simulink model "NUgus_contact"  (R2018a)
settings: Solver=VariableStepAuto  StartTime=0.0  StopTime=inf  RelTol=1e-3
values from neighbouring files (symbols this model uses):
  h_pitch = 0    [init.m]    (also in zombie.m)
  h_yaw = 0    [init.m]    (also in zombie.m)
  head = [-0.05482228998067195, -0.00010888238321339966, 0.0011712900228573724, 0.41900000000000004]    [comtest.m]
  l_ankle_pitch = 0    [init.m]    (also in zombie.m)
  l_ankle_roll = 0    [init.m]    (also in zombie.m)
  l_elbow_pitch = 0    [init.m]    (also in zombie.m)
  l_hip_pitch = 0    [init.m]    (also in zombie.m)
  l_hip_roll = 0    [init.m]    (also in zombie.m)
  l_hip_yaw = 0    [init.m]    (also in zombie.m)
  l_knee_pitch = 0    [init.m]    (also in zombie.m)
  l_shoulder_pitch = 0    [init.m]    (also in zombie.m)
  l_shoulder_roll = 0    [init.m]    (also in zombie.m)
  r_ankle_pitch = 0    [init.m]    (also in zombie.m)
  r_ankle_roll = 0    [init.m]    (also in zombie.m)
  r_elbow_pitch = 0    [init.m]    (also in zombie.m)
  r_hip_pitch = 0    [init.m]    (also in zombie.m)
  r_hip_roll = 0    [init.m]    (also in zombie.m)
  r_hip_yaw = 0    [init.m]    (also in zombie.m)
  r_knee_pitch = 0    [init.m]    (also in zombie.m)
  r_shoulder_pitch = 0    [init.m]    (also in zombie.m)
  r_shoulder_roll = 0    [init.m]    (also in zombie.m)
  s = mean(abs(present_speed.data))    [RunServoTest.m]
  torso = [0.0050079703254699804, 0.008880921777563762, 0.1021503146237477, 2.5390000000000006]    [comtest.m]
undefined symbols (not defined in the file or in its folder): floor, X, Y, Z
libraries: sm_lib x206, fl_lib x128, nesl_utility x21
(part 6 of 6)

== system NUgus_contact/right_foot/foot_fr_contact ==
  6-DOF Joint : sm_lib/Joints/6-DOF Joint  SenseConstraintForce=off  SenseConstraintForceX=off  SenseConstraintForceY=off  SenseConstraintForceZ=off  SenseConstraintTorque=off  SenseConstraintTorqueX=off  SenseConstraintTorqueY=off  SenseConstraintTorqueZ=off  SenseTotalForce=off  SenseTotalForceX=off  SenseTotalForceY=off  SenseTotalForceZ=off  SenseTotalTorque=off  SenseTotalTorqueX=off  SenseTotalTorqueY=off  SenseTotalTorqueZ=off  CompositeWrenchDir=FollowerOnBase  CompositeWrenchFrame=BaseFrame  PxEquilibriumPosition=0  PxEquilibriumPositionUnits=m  PxSpringStiffness=0  PxSpringStiffnessUnits=N/m  PxDampingCoefficient=0  PxDampingCoefficientUnits=N/(m/s)  PxTorqueActuationMode=InputTorque  PxMotionActuationMode=ComputedMotion  PxSensePosition=off  PxSenseVelocity=on  PxSenseAcceleration=off  PxSenseTorqueForce=off  PxPositionTargetSpecify=off  PxPositionTargetPriority=High  PxPositionTargetValue=0  PxPositionTargetValueUnits=m  PxVelocityTargetSpecify=off  PxVelocityTargetPriority=High  PxVelocityTargetValue=0  PxVelocityTargetValueUnits=m/s  PyEquilibriumPosition=0  PyEquilibriumPositionUnits=m  PySpringStiffness=0  PySpringStiffnessUnits=N/m  PyDampingCoefficient=0  PyDampingCoefficientUnits=N/(m/s)  PyTorqueActuationMode=InputTorque  PyMotionActuationMode=ComputedMotion  PySensePosition=off  PySenseVelocity=on  PySenseAcceleration=off  PySenseTorqueForce=off  PyPositionTargetSpecify=off  PyPositionTargetPriority=High  PyPositionTargetValue=0  PyPositionTargetValueUnits=m  PyVelocityTargetSpecify=off  PyVelocityTargetPriority=High  PyVelocityTargetValue=0  PyVelocityTargetValueUnits=m/s  PzEquilibriumPosition=0  PzEquilibriumPositionUnits=m  PzSpringStiffness=0  PzSpringStiffnessUnits=N/m  PzDampingCoefficient=0  PzDampingCoefficientUnits=N/(m/s)  PzTorqueActuationMode=InputTorque  PzMotionActuationMode=ComputedMotion  PzSensePosition=on  PzSenseVelocity=on  PzSenseAcceleration=off  PzSenseTorqueForce=off  PzPositionTargetSpecify=off  PzPositionTargetPriority=High  PzPositionTargetValue=0  PzPositionTargetValueUnits=m  PzVelocityTargetSpecify=off  PzVelocityTargetPriority=High  PzVelocityTargetValue=0  PzVelocityTargetValueUnits=m/s  SphDefPosRotationMethod=None  SphDefPosRotationAngleUnits=deg  SphDefPosRotationStandardAxis=+Z  SphDefPosRotationAngle=0.0  SphDefPosRotationArbitraryAxis=[0 0 1]  SphDefPosFollAlignAxisA=+X  SphDefPosBaseAlignAxisA=+Y  SphDefPosFollAlignAxisB=+Y  SphDefPosBaseAlignAxisB=+Z  SphDefPosRotationSequenceAxes=FollowerAxes  SphDefPosRotationSequence=XYX  SphDefPosRotationSequenceAngles=[0 0 0]  SphDefPosRotationSequenceAnglesUnits=deg  SphDefPosRotationMatrix=[1 0 0; 0 1 0; 0 0 1]  SphEqPosRotationMethod=None  SphEqPosRotationAngleUnits=deg  SphEqPosRotationStandardAxis=+Z  SphEqPosRotationAngle=0.0  SphEqPosRotationArbitraryAxis=[0 0 1]  SphEqPosFollAlignAxisA=+X  SphEqPosBaseAlignAxisA=+Y  SphEqPosFollAlignAxisB=+Y  SphEqPosBaseAlignAxisB=+Z  SphEqPosRotationSequenceAxes=FollowerAxes  SphEqPosRotationSequence=XYX  SphEqPosRotationSequenceAngles=[0 0 0]  SphEqPosRotationSequenceAnglesUnits=deg  SphEqPosRotationMatrix=[1 0 0; 0 1 0; 0 0 1]  SphSpringStiffness=0  SphSpringStiffnessUnits=N*m/deg  SphDampingCoefficient=0  SphDampingCoefficientUnits=N*m/(deg/s)  SphActuateTorqueX=off  SphActuateTorqueY=off  SphActuateTorqueZ=off  SphActuateTorque=off  SphTorqueActuationMode=NoTorque  SphMotionActuationMode=ComputedMotion  SphActuationFrame=BaseFrame  SphSensePosition=off  SphSenseVelocityX=off  SphSenseVelocityY=off  SphSenseVelocityZ=off  SphSenseVelocity=off  SphSenseAccelerationX=off  SphSenseAccelerationY=off  SphSenseAccelerationZ=off  SphSenseAcceleration=off  SphSenseTorqueX=off  SphSenseTorqueY=off  SphSenseTorqueZ=off  SphSenseTorqueForce=off  SphSensingFrame=BaseFrame  SphPositionTargetRotationMethod=None  SphPositionTargetRotationAngleUnits=deg  SphPositionTargetRotationStandardAxis=+Z  SphPositionTargetRotationAngle=0.0  SphPositionTargetRotationArbitraryAxis=[0 0 1]  SphPositionTargetFollAlignAxisA=+X  SphPositionTargetBaseAlignAxisA=+Y  SphPositionTargetFollAlignAxisB=+Y  SphPositionTargetBaseAlignAxisB=+Z  SphPositionTargetRotationSequenceAxes=FollowerAxes  SphPositionTargetRotationSequence=XYX  SphPositionTargetRotationSequenceAngles=[0 0 0]  SphPositionTargetRotationSequenceAnglesUnits=deg  SphPositionTargetRotationMatrix=[1 0 0; 0 1 0; 0 0 1]  SphPositionTargetSpecify=off  SphPositionTargetPriority=High  SphVelocityTargetValue=[0 0 0]  SphVelocityTargetValueUnits=deg/s  SphVelocityTargetSpecify=off  SphVelocityTargetPriority=High  SphVelocityTargetInFollowerFrame=on
  PS Abs : fl_lib/Physical Signals/Nonlinear Operators/PS Abs
      settings: SourceProductName=Simscape  SourceProductBaseCode=SS
  calculate forces : Subsystem
  friction gain : fl_lib/Physical Signals/Functions/PS Gain  gain=floor.friction
  x Velocity Gain : fl_lib/Physical Signals/Functions/PS Gain  gain=floor.vel_gain
  y Velocity Gain : fl_lib/Physical Signals/Functions/PS Gain  gain=floor.vel_gain
  z Position gain : fl_lib/Physical Signals/Functions/PS Gain  gain=floor.pos_gain
  z Velocity Gain : fl_lib/Physical Signals/Functions/PS Gain  gain=floor.vel_gain
  z add : fl_lib/Physical Signals/Functions/PS Add
  Contact : PMIOPort  Side=Right
  Floor : PMIOPort  Port=2  Side=Left
  connections:
  6-DOF Joint/RConn1 -- Contact/RConn1
  Floor/RConn1 -- 6-DOF Joint/LConn1
  6-DOF Joint/RConn4 -- calculate forces/LConn3 -- z Position gain/LConn1
  z Velocity Gain/LConn1 -- 6-DOF Joint/RConn5
  y Velocity Gain/LConn1 -- 6-DOF Joint/RConn3
  x Velocity Gain/LConn1 -- 6-DOF Joint/RConn2
  z Position gain/RConn1 -- z add/LConn1
  z Velocity Gain/RConn1 -- z add/LConn2
  PS Abs/LConn1 -- friction gain/RConn1
  z add/RConn1 -- friction gain/LConn1 -- calculate forces/LConn4
  calculate forces/LConn1 -- x Velocity Gain/RConn1
  calculate forces/LConn2 -- y Velocity Gain/RConn1
  calculate forces/LConn5 -- PS Abs/RConn1
  calculate forces/RConn1 -- 6-DOF Joint/LConn2
  calculate forces/RConn2 -- 6-DOF Joint/LConn3
  calculate forces/RConn3 -- 6-DOF Joint/LConn4

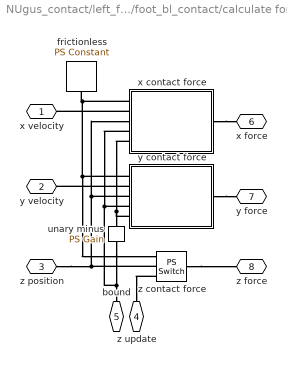
== system NUgus_contact/left_foot/foot_bl_contact/calculate forces ==
  frictionless : fl_lib/Physical Signals/Sources/PS Constant  constant=0
  unary minus : fl_lib/Physical Signals/Functions/PS Gain  gain=-1
  x contact force : Subsystem
  y contact force : Subsystem
  z contact force : fl_lib/Physical Signals/Nonlinear Operators/PS Switch  Threshold=0
      settings: SourceProductName=Simscape  SourceProductBaseCode=SS
  x velocity : PMIOPort  Side=Left
  y velocity : PMIOPort  Port=2  Side=Left
  z position : PMIOPort  Port=3  Side=Left
  z update : PMIOPort  Port=4  Side=Left
  bound : PMIOPort  Port=5  Side=Left
  x force : PMIOPort  Port=6  Side=Right
  y force : PMIOPort  Port=7  Side=Right
  z force : PMIOPort  Port=8  Side=Right
  connections:
  x contact force/LConn2 -- x velocity/RConn1
  y contact force/LConn2 -- y velocity/RConn1
  y contact force/RConn1 -- y force/RConn1
  x contact force/RConn1 -- x force/RConn1
  z contact force/RConn1 -- z force/RConn1
  y contact force/LConn3 -- x contact force/LConn3 -- z position/RConn1 -- z contact force/LConn2
  y contact force/LConn4 -- x contact force/LConn4 -- unary minus/LConn1 -- bound/RConn1
  y contact force/LConn5 -- x contact force/LConn5 -- unary minus/RConn1
  x contact force/LConn1 -- frictionless/RConn1 -- y contact force/LConn1 -- z contact force/LConn1
  z contact force/LConn3 -- z update/RConn1

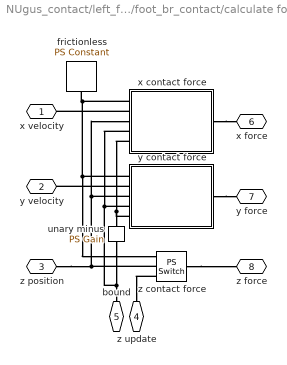
== system NUgus_contact/left_foot/foot_br_contact/calculate forces ==
  frictionless : fl_lib/Physical Signals/Sources/PS Constant  constant=0
  unary minus : fl_lib/Physical Signals/Functions/PS Gain  gain=-1
  x contact force : Subsystem
  y contact force : Subsystem
  z contact force : fl_lib/Physical Signals/Nonlinear Operators/PS Switch  Threshold=0
      settings: SourceProductName=Simscape  SourceProductBaseCode=SS
  x velocity : PMIOPort  Side=Left
  y velocity : PMIOPort  Port=2  Side=Left
  z position : PMIOPort  Port=3  Side=Left
  z update : PMIOPort  Port=4  Side=Left
  bound : PMIOPort  Port=5  Side=Left
  x force : PMIOPort  Port=6  Side=Right
  y force : PMIOPort  Port=7  Side=Right
  z force : PMIOPort  Port=8  Side=Right
  connections:
  x contact force/LConn2 -- x velocity/RConn1
  y contact force/LConn2 -- y velocity/RConn1
  y contact force/RConn1 -- y force/RConn1
  x contact force/RConn1 -- x force/RConn1
  z contact force/RConn1 -- z force/RConn1
  y contact force/LConn3 -- x contact force/LConn3 -- z position/RConn1 -- z contact force/LConn2
  y contact force/LConn4 -- x contact force/LConn4 -- unary minus/LConn1 -- bound/RConn1
  y contact force/LConn5 -- x contact force/LConn5 -- unary minus/RConn1
  x contact force/LConn1 -- frictionless/RConn1 -- y contact force/LConn1 -- z contact force/LConn1
  z contact force/LConn3 -- z update/RConn1

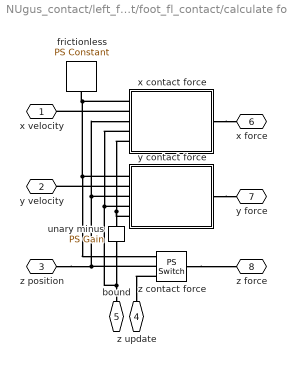
== system NUgus_contact/left_foot/foot_fl_contact/calculate forces ==
  frictionless : fl_lib/Physical Signals/Sources/PS Constant  constant=0
  unary minus : fl_lib/Physical Signals/Functions/PS Gain  gain=-1
  x contact force : Subsystem
  y contact force : Subsystem
  z contact force : fl_lib/Physical Signals/Nonlinear Operators/PS Switch  Threshold=0
      settings: SourceProductName=Simscape  SourceProductBaseCode=SS
  x velocity : PMIOPort  Side=Left
  y velocity : PMIOPort  Port=2  Side=Left
  z position : PMIOPort  Port=3  Side=Left
  z update : PMIOPort  Port=4  Side=Left
  bound : PMIOPort  Port=5  Side=Left
  x force : PMIOPort  Port=6  Side=Right
  y force : PMIOPort  Port=7  Side=Right
  z force : PMIOPort  Port=8  Side=Right
  connections:
  x contact force/LConn2 -- x velocity/RConn1
  y contact force/LConn2 -- y velocity/RConn1
  y contact force/RConn1 -- y force/RConn1
  x contact force/RConn1 -- x force/RConn1
  z contact force/RConn1 -- z force/RConn1
  y contact force/LConn3 -- x contact force/LConn3 -- z position/RConn1 -- z contact force/LConn2
  y contact force/LConn4 -- x contact force/LConn4 -- unary minus/LConn1 -- bound/RConn1
  y contact force/LConn5 -- x contact force/LConn5 -- unary minus/RConn1
  x contact force/LConn1 -- frictionless/RConn1 -- y contact force/LConn1 -- z contact force/LConn1
  z contact force/LConn3 -- z update/RConn1

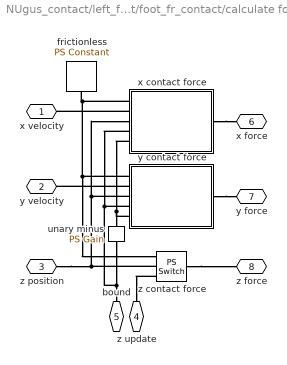
== system NUgus_contact/left_foot/foot_fr_contact/calculate forces ==
  frictionless : fl_lib/Physical Signals/Sources/PS Constant  constant=0
  unary minus : fl_lib/Physical Signals/Functions/PS Gain  gain=-1
  x contact force : Subsystem
  y contact force : Subsystem
  z contact force : fl_lib/Physical Signals/Nonlinear Operators/PS Switch  Threshold=0
      settings: SourceProductName=Simscape  SourceProductBaseCode=SS
  x velocity : PMIOPort  Side=Left
  y velocity : PMIOPort  Port=2  Side=Left
  z position : PMIOPort  Port=3  Side=Left
  z update : PMIOPort  Port=4  Side=Left
  bound : PMIOPort  Port=5  Side=Left
  x force : PMIOPort  Port=6  Side=Right
  y force : PMIOPort  Port=7  Side=Right
  z force : PMIOPort  Port=8  Side=Right
  connections:
  x contact force/LConn2 -- x velocity/RConn1
  y contact force/LConn2 -- y velocity/RConn1
  y contact force/RConn1 -- y force/RConn1
  x contact force/RConn1 -- x force/RConn1
  z contact force/RConn1 -- z force/RConn1
  y contact force/LConn3 -- x contact force/LConn3 -- z position/RConn1 -- z contact force/LConn2
  y contact force/LConn4 -- x contact force/LConn4 -- unary minus/LConn1 -- bound/RConn1
  y contact force/LConn5 -- x contact force/LConn5 -- unary minus/RConn1
  x contact force/LConn1 -- frictionless/RConn1 -- y contact force/LConn1 -- z contact force/LConn1
  z contact force/LConn3 -- z update/RConn1

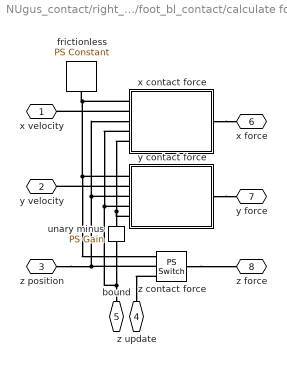
== system NUgus_contact/right_foot/foot_bl_contact/calculate forces ==
  frictionless : fl_lib/Physical Signals/Sources/PS Constant  constant=0
  unary minus : fl_lib/Physical Signals/Functions/PS Gain  gain=-1
  x contact force : Subsystem
  y contact force : Subsystem
  z contact force : fl_lib/Physical Signals/Nonlinear Operators/PS Switch  Threshold=0
      settings: SourceProductName=Simscape  SourceProductBaseCode=SS
  x velocity : PMIOPort  Side=Left
  y velocity : PMIOPort  Port=2  Side=Left
  z position : PMIOPort  Port=3  Side=Left
  z update : PMIOPort  Port=4  Side=Left
  bound : PMIOPort  Port=5  Side=Left
  x force : PMIOPort  Port=6  Side=Right
  y force : PMIOPort  Port=7  Side=Right
  z force : PMIOPort  Port=8  Side=Right
  connections:
  x contact force/LConn2 -- x velocity/RConn1
  y contact force/LConn2 -- y velocity/RConn1
  y contact force/RConn1 -- y force/RConn1
  x contact force/RConn1 -- x force/RConn1
  z contact force/RConn1 -- z force/RConn1
  y contact force/LConn3 -- x contact force/LConn3 -- z position/RConn1 -- z contact force/LConn2
  y contact force/LConn4 -- x contact force/LConn4 -- unary minus/LConn1 -- bound/RConn1
  y contact force/LConn5 -- x contact force/LConn5 -- unary minus/RConn1
  x contact force/LConn1 -- frictionless/RConn1 -- y contact force/LConn1 -- z contact force/LConn1
  z contact force/LConn3 -- z update/RConn1

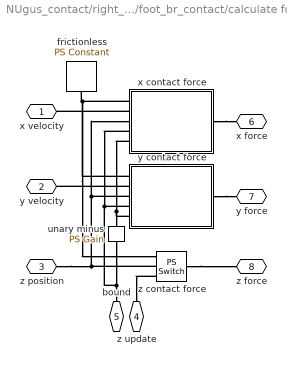
== system NUgus_contact/right_foot/foot_br_contact/calculate forces ==
  frictionless : fl_lib/Physical Signals/Sources/PS Constant  constant=0
  unary minus : fl_lib/Physical Signals/Functions/PS Gain  gain=-1
  x contact force : Subsystem
  y contact force : Subsystem
  z contact force : fl_lib/Physical Signals/Nonlinear Operators/PS Switch  Threshold=0
      settings: SourceProductName=Simscape  SourceProductBaseCode=SS
  x velocity : PMIOPort  Side=Left
  y velocity : PMIOPort  Port=2  Side=Left
  z position : PMIOPort  Port=3  Side=Left
  z update : PMIOPort  Port=4  Side=Left
  bound : PMIOPort  Port=5  Side=Left
  x force : PMIOPort  Port=6  Side=Right
  y force : PMIOPort  Port=7  Side=Right
  z force : PMIOPort  Port=8  Side=Right
  connections:
  x contact force/LConn2 -- x velocity/RConn1
  y contact force/LConn2 -- y velocity/RConn1
  y contact force/RConn1 -- y force/RConn1
  x contact force/RConn1 -- x force/RConn1
  z contact force/RConn1 -- z force/RConn1
  z contact force/LConn2 -- z position/RConn1 -- y contact force/LConn3 -- x contact force/LConn3
  unary minus/LConn1 -- y contact force/LConn4 -- x contact force/LConn4 -- bound/RConn1
  x contact force/LConn5 -- y contact force/LConn5 -- unary minus/RConn1
  x contact force/LConn1 -- y contact force/LConn1 -- z contact force/LConn1 -- frictionless/RConn1
  z contact force/LConn3 -- z update/RConn1

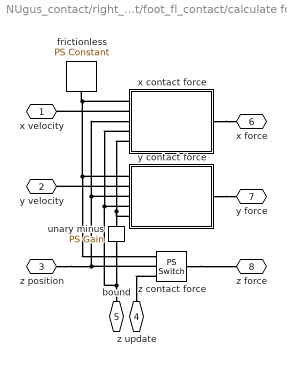
== system NUgus_contact/right_foot/foot_fl_contact/calculate forces ==
  frictionless : fl_lib/Physical Signals/Sources/PS Constant  constant=0
  unary minus : fl_lib/Physical Signals/Functions/PS Gain  gain=-1
  x contact force : Subsystem
  y contact force : Subsystem
  z contact force : fl_lib/Physical Signals/Nonlinear Operators/PS Switch  Threshold=0
      settings: SourceProductName=Simscape  SourceProductBaseCode=SS
  x velocity : PMIOPort  Side=Left
  y velocity : PMIOPort  Port=2  Side=Left
  z position : PMIOPort  Port=3  Side=Left
  z update : PMIOPort  Port=4  Side=Left
  bound : PMIOPort  Port=5  Side=Left
  x force : PMIOPort  Port=6  Side=Right
  y force : PMIOPort  Port=7  Side=Right
  z force : PMIOPort  Port=8  Side=Right
  connections:
  x contact force/LConn2 -- x velocity/RConn1
  y contact force/LConn2 -- y velocity/RConn1
  y contact force/RConn1 -- y force/RConn1
  x contact force/RConn1 -- x force/RConn1
  z contact force/RConn1 -- z force/RConn1
  y contact force/LConn3 -- x contact force/LConn3 -- z position/RConn1 -- z contact force/LConn2
  y contact force/LConn4 -- x contact force/LConn4 -- unary minus/LConn1 -- bound/RConn1
  y contact force/LConn5 -- x contact force/LConn5 -- unary minus/RConn1
  x contact force/LConn1 -- frictionless/RConn1 -- y contact force/LConn1 -- z contact force/LConn1
  z contact force/LConn3 -- z update/RConn1

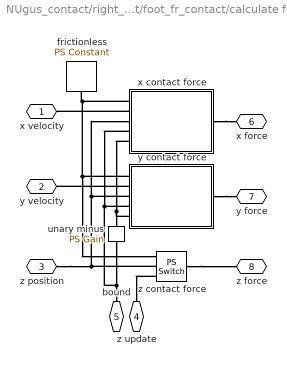
== system NUgus_contact/right_foot/foot_fr_contact/calculate forces ==
  frictionless : fl_lib/Physical Signals/Sources/PS Constant  constant=0
  unary minus : fl_lib/Physical Signals/Functions/PS Gain  gain=-1
  x contact force : Subsystem
  y contact force : Subsystem
  z contact force : fl_lib/Physical Signals/Nonlinear Operators/PS Switch  Threshold=0
      settings: SourceProductName=Simscape  SourceProductBaseCode=SS
  x velocity : PMIOPort  Side=Left
  y velocity : PMIOPort  Port=2  Side=Left
  z position : PMIOPort  Port=3  Side=Left
  z update : PMIOPort  Port=4  Side=Left
  bound : PMIOPort  Port=5  Side=Left
  x force : PMIOPort  Port=6  Side=Right
  y force : PMIOPort  Port=7  Side=Right
  z force : PMIOPort  Port=8  Side=Right
  connections:
  x contact force/LConn2 -- x velocity/RConn1
  y contact force/LConn2 -- y velocity/RConn1
  y contact force/RConn1 -- y force/RConn1
  x contact force/RConn1 -- x force/RConn1
  z contact force/RConn1 -- z force/RConn1
  y contact force/LConn3 -- x contact force/LConn3 -- z position/RConn1 -- z contact force/LConn2
  y contact force/LConn4 -- x contact force/LConn4 -- unary minus/LConn1 -- bound/RConn1
  y contact force/LConn5 -- x contact force/LConn5 -- unary minus/RConn1
  x contact force/LConn1 -- frictionless/RConn1 -- y contact force/LConn1 -- z contact force/LConn1
  z contact force/LConn3 -- z update/RConn1

== system NUgus_contact/left_foot/foot_bl_contact/calculate forces/x contact force ==
  PS Max : fl_lib/Physical Signals/Nonlinear Operators/PS Max
      settings: SourceProductName=Simscape  SourceProductBaseCode=SS
  PS Min : fl_lib/Physical Signals/Nonlinear Operators/PS Min
      settings: SourceProductName=Simscape  SourceProductBaseCode=SS
  PS Switch1 : fl_lib/Physical Signals/Nonlinear Operators/PS Switch  Threshold=0
      settings: SourceProductName=Simscape  SourceProductBaseCode=SS
  frictionless : PMIOPort  Side=Left
  force : PMIOPort  Port=2  Side=Right
  velocity : PMIOPort  Port=3  Side=Left
  z position : PMIOPort  Port=4  Side=Left
  upper_bound : PMIOPort  Port=5  Side=Left
  lower_bound : PMIOPort  Port=6  Side=Left
  connections:
  PS Max/LConn2 -- lower_bound/RConn1
  PS Max/LConn1 -- PS Min/RConn1
  PS Switch1/LConn3 -- PS Max/RConn1
  PS Min/LConn1 -- velocity/RConn1
  z position/RConn1 -- PS Switch1/LConn2
  PS Switch1/LConn1 -- frictionless/RConn1
  PS Switch1/RConn1 -- force/RConn1
  PS Min/LConn2 -- upper_bound/RConn1

== system NUgus_contact/left_foot/foot_bl_contact/calculate forces/y contact force ==
  PS Max : fl_lib/Physical Signals/Nonlinear Operators/PS Max
      settings: SourceProductName=Simscape  SourceProductBaseCode=SS
  PS Min : fl_lib/Physical Signals/Nonlinear Operators/PS Min
      settings: SourceProductName=Simscape  SourceProductBaseCode=SS
  PS Switch1 : fl_lib/Physical Signals/Nonlinear Operators/PS Switch  Threshold=0
      settings: SourceProductName=Simscape  SourceProductBaseCode=SS
  frictionless : PMIOPort  Side=Left
  force : PMIOPort  Port=2  Side=Right
  velocity : PMIOPort  Port=3  Side=Left
  z position : PMIOPort  Port=4  Side=Left
  upper_bound : PMIOPort  Port=5  Side=Left
  lower_bound : PMIOPort  Port=6  Side=Left
  connections:
  PS Max/LConn2 -- lower_bound/RConn1
  PS Max/LConn1 -- PS Min/RConn1
  PS Switch1/LConn3 -- PS Max/RConn1
  PS Min/LConn1 -- velocity/RConn1
  z position/RConn1 -- PS Switch1/LConn2
  PS Switch1/LConn1 -- frictionless/RConn1
  PS Switch1/RConn1 -- force/RConn1
  PS Min/LConn2 -- upper_bound/RConn1

== system NUgus_contact/left_foot/foot_br_contact/calculate forces/x contact force ==
  PS Max : fl_lib/Physical Signals/Nonlinear Operators/PS Max
      settings: SourceProductName=Simscape  SourceProductBaseCode=SS
  PS Min : fl_lib/Physical Signals/Nonlinear Operators/PS Min
      settings: SourceProductName=Simscape  SourceProductBaseCode=SS
  PS Switch1 : fl_lib/Physical Signals/Nonlinear Operators/PS Switch  Threshold=0
      settings: SourceProductName=Simscape  SourceProductBaseCode=SS
  frictionless : PMIOPort  Side=Left
  force : PMIOPort  Port=2  Side=Right
  velocity : PMIOPort  Port=3  Side=Left
  z position : PMIOPort  Port=4  Side=Left
  upper_bound : PMIOPort  Port=5  Side=Left
  lower_bound : PMIOPort  Port=6  Side=Left
  connections:
  PS Max/LConn2 -- lower_bound/RConn1
  PS Max/LConn1 -- PS Min/RConn1
  PS Switch1/LConn3 -- PS Max/RConn1
  PS Min/LConn1 -- velocity/RConn1
  z position/RConn1 -- PS Switch1/LConn2
  PS Switch1/LConn1 -- frictionless/RConn1
  PS Switch1/RConn1 -- force/RConn1
  PS Min/LConn2 -- upper_bound/RConn1

== system NUgus_contact/left_foot/foot_br_contact/calculate forces/y contact force ==
  PS Max : fl_lib/Physical Signals/Nonlinear Operators/PS Max
      settings: SourceProductName=Simscape  SourceProductBaseCode=SS
  PS Min : fl_lib/Physical Signals/Nonlinear Operators/PS Min
      settings: SourceProductName=Simscape  SourceProductBaseCode=SS
  PS Switch1 : fl_lib/Physical Signals/Nonlinear Operators/PS Switch  Threshold=0
      settings: SourceProductName=Simscape  SourceProductBaseCode=SS
  frictionless : PMIOPort  Side=Left
  force : PMIOPort  Port=2  Side=Right
  velocity : PMIOPort  Port=3  Side=Left
  z position : PMIOPort  Port=4  Side=Left
  upper_bound : PMIOPort  Port=5  Side=Left
  lower_bound : PMIOPort  Port=6  Side=Left
  connections:
  PS Max/LConn2 -- lower_bound/RConn1
  PS Max/LConn1 -- PS Min/RConn1
  PS Switch1/LConn3 -- PS Max/RConn1
  PS Min/LConn1 -- velocity/RConn1
  z position/RConn1 -- PS Switch1/LConn2
  PS Switch1/LConn1 -- frictionless/RConn1
  PS Switch1/RConn1 -- force/RConn1
  PS Min/LConn2 -- upper_bound/RConn1

== system NUgus_contact/left_foot/foot_fl_contact/calculate forces/x contact force ==
  PS Max : fl_lib/Physical Signals/Nonlinear Operators/PS Max
      settings: SourceProductName=Simscape  SourceProductBaseCode=SS
  PS Min : fl_lib/Physical Signals/Nonlinear Operators/PS Min
      settings: SourceProductName=Simscape  SourceProductBaseCode=SS
  PS Switch1 : fl_lib/Physical Signals/Nonlinear Operators/PS Switch  Threshold=0
      settings: SourceProductName=Simscape  SourceProductBaseCode=SS
  frictionless : PMIOPort  Side=Left
  force : PMIOPort  Port=2  Side=Right
  velocity : PMIOPort  Port=3  Side=Left
  z position : PMIOPort  Port=4  Side=Left
  upper_bound : PMIOPort  Port=5  Side=Left
  lower_bound : PMIOPort  Port=6  Side=Left
  connections:
  PS Max/LConn2 -- lower_bound/RConn1
  PS Max/LConn1 -- PS Min/RConn1
  PS Switch1/LConn3 -- PS Max/RConn1
  PS Min/LConn1 -- velocity/RConn1
  z position/RConn1 -- PS Switch1/LConn2
  PS Switch1/LConn1 -- frictionless/RConn1
  PS Switch1/RConn1 -- force/RConn1
  PS Min/LConn2 -- upper_bound/RConn1

== system NUgus_contact/left_foot/foot_fl_contact/calculate forces/y contact force ==
  PS Max : fl_lib/Physical Signals/Nonlinear Operators/PS Max
      settings: SourceProductName=Simscape  SourceProductBaseCode=SS
  PS Min : fl_lib/Physical Signals/Nonlinear Operators/PS Min
      settings: SourceProductName=Simscape  SourceProductBaseCode=SS
  PS Switch1 : fl_lib/Physical Signals/Nonlinear Operators/PS Switch  Threshold=0
      settings: SourceProductName=Simscape  SourceProductBaseCode=SS
  frictionless : PMIOPort  Side=Left
  force : PMIOPort  Port=2  Side=Right
  velocity : PMIOPort  Port=3  Side=Left
  z position : PMIOPort  Port=4  Side=Left
  upper_bound : PMIOPort  Port=5  Side=Left
  lower_bound : PMIOPort  Port=6  Side=Left
  connections:
  PS Max/LConn2 -- lower_bound/RConn1
  PS Max/LConn1 -- PS Min/RConn1
  PS Switch1/LConn3 -- PS Max/RConn1
  PS Min/LConn1 -- velocity/RConn1
  z position/RConn1 -- PS Switch1/LConn2
  PS Switch1/LConn1 -- frictionless/RConn1
  PS Switch1/RConn1 -- force/RConn1
  PS Min/LConn2 -- upper_bound/RConn1

== system NUgus_contact/left_foot/foot_fr_contact/calculate forces/x contact force ==
  PS Max : fl_lib/Physical Signals/Nonlinear Operators/PS Max
      settings: SourceProductName=Simscape  SourceProductBaseCode=SS
  PS Min : fl_lib/Physical Signals/Nonlinear Operators/PS Min
      settings: SourceProductName=Simscape  SourceProductBaseCode=SS
  PS Switch1 : fl_lib/Physical Signals/Nonlinear Operators/PS Switch  Threshold=0
      settings: SourceProductName=Simscape  SourceProductBaseCode=SS
  frictionless : PMIOPort  Side=Left
  force : PMIOPort  Port=2  Side=Right
  velocity : PMIOPort  Port=3  Side=Left
  z position : PMIOPort  Port=4  Side=Left
  upper_bound : PMIOPort  Port=5  Side=Left
  lower_bound : PMIOPort  Port=6  Side=Left
  connections:
  PS Max/LConn2 -- lower_bound/RConn1
  PS Max/LConn1 -- PS Min/RConn1
  PS Switch1/LConn3 -- PS Max/RConn1
  PS Min/LConn1 -- velocity/RConn1
  z position/RConn1 -- PS Switch1/LConn2
  PS Switch1/LConn1 -- frictionless/RConn1
  PS Switch1/RConn1 -- force/RConn1
  PS Min/LConn2 -- upper_bound/RConn1

== system NUgus_contact/left_foot/foot_fr_contact/calculate forces/y contact force ==
  PS Max : fl_lib/Physical Signals/Nonlinear Operators/PS Max
      settings: SourceProductName=Simscape  SourceProductBaseCode=SS
  PS Min : fl_lib/Physical Signals/Nonlinear Operators/PS Min
      settings: SourceProductName=Simscape  SourceProductBaseCode=SS
  PS Switch1 : fl_lib/Physical Signals/Nonlinear Operators/PS Switch  Threshold=0
      settings: SourceProductName=Simscape  SourceProductBaseCode=SS
  frictionless : PMIOPort  Side=Left
  force : PMIOPort  Port=2  Side=Right
  velocity : PMIOPort  Port=3  Side=Left
  z position : PMIOPort  Port=4  Side=Left
  upper_bound : PMIOPort  Port=5  Side=Left
  lower_bound : PMIOPort  Port=6  Side=Left
  connections:
  PS Max/LConn2 -- lower_bound/RConn1
  PS Max/LConn1 -- PS Min/RConn1
  PS Switch1/LConn3 -- PS Max/RConn1
  PS Min/LConn1 -- velocity/RConn1
  z position/RConn1 -- PS Switch1/LConn2
  PS Switch1/LConn1 -- frictionless/RConn1
  PS Switch1/RConn1 -- force/RConn1
  PS Min/LConn2 -- upper_bound/RConn1

== system NUgus_contact/right_foot/foot_bl_contact/calculate forces/x contact force ==
  PS Max : fl_lib/Physical Signals/Nonlinear Operators/PS Max
      settings: SourceProductName=Simscape  SourceProductBaseCode=SS
  PS Min : fl_lib/Physical Signals/Nonlinear Operators/PS Min
      settings: SourceProductName=Simscape  SourceProductBaseCode=SS
  PS Switch1 : fl_lib/Physical Signals/Nonlinear Operators/PS Switch  Threshold=0
      settings: SourceProductName=Simscape  SourceProductBaseCode=SS
  frictionless : PMIOPort  Side=Left
  force : PMIOPort  Port=2  Side=Right
  velocity : PMIOPort  Port=3  Side=Left
  z position : PMIOPort  Port=4  Side=Left
  upper_bound : PMIOPort  Port=5  Side=Left
  lower_bound : PMIOPort  Port=6  Side=Left
  connections:
  PS Max/LConn2 -- lower_bound/RConn1
  PS Max/LConn1 -- PS Min/RConn1
  PS Switch1/LConn3 -- PS Max/RConn1
  PS Min/LConn1 -- velocity/RConn1
  z position/RConn1 -- PS Switch1/LConn2
  PS Switch1/LConn1 -- frictionless/RConn1
  PS Switch1/RConn1 -- force/RConn1
  PS Min/LConn2 -- upper_bound/RConn1

== system NUgus_contact/right_foot/foot_bl_contact/calculate forces/y contact force ==
  PS Max : fl_lib/Physical Signals/Nonlinear Operators/PS Max
      settings: SourceProductName=Simscape  SourceProductBaseCode=SS
  PS Min : fl_lib/Physical Signals/Nonlinear Operators/PS Min
      settings: SourceProductName=Simscape  SourceProductBaseCode=SS
  PS Switch1 : fl_lib/Physical Signals/Nonlinear Operators/PS Switch  Threshold=0
      settings: SourceProductName=Simscape  SourceProductBaseCode=SS
  frictionless : PMIOPort  Side=Left
  force : PMIOPort  Port=2  Side=Right
  velocity : PMIOPort  Port=3  Side=Left
  z position : PMIOPort  Port=4  Side=Left
  upper_bound : PMIOPort  Port=5  Side=Left
  lower_bound : PMIOPort  Port=6  Side=Left
  connections:
  PS Max/LConn2 -- lower_bound/RConn1
  PS Max/LConn1 -- PS Min/RConn1
  PS Switch1/LConn3 -- PS Max/RConn1
  PS Min/LConn1 -- velocity/RConn1
  z position/RConn1 -- PS Switch1/LConn2
  PS Switch1/LConn1 -- frictionless/RConn1
  PS Switch1/RConn1 -- force/RConn1
  PS Min/LConn2 -- upper_bound/RConn1

== system NUgus_contact/right_foot/foot_br_contact/calculate forces/x contact force ==
  PS Max : fl_lib/Physical Signals/Nonlinear Operators/PS Max
      settings: SourceProductName=Simscape  SourceProductBaseCode=SS
  PS Min : fl_lib/Physical Signals/Nonlinear Operators/PS Min
      settings: SourceProductName=Simscape  SourceProductBaseCode=SS
  PS Switch1 : fl_lib/Physical Signals/Nonlinear Operators/PS Switch  Threshold=0
      settings: SourceProductName=Simscape  SourceProductBaseCode=SS
  frictionless : PMIOPort  Side=Left
  force : PMIOPort  Port=2  Side=Right
  velocity : PMIOPort  Port=3  Side=Left
  z position : PMIOPort  Port=4  Side=Left
  upper_bound : PMIOPort  Port=5  Side=Left
  lower_bound : PMIOPort  Port=6  Side=Left
  connections:
  PS Max/LConn2 -- lower_bound/RConn1
  PS Max/LConn1 -- PS Min/RConn1
  PS Switch1/LConn3 -- PS Max/RConn1
  PS Min/LConn1 -- velocity/RConn1
  z position/RConn1 -- PS Switch1/LConn2
  PS Switch1/LConn1 -- frictionless/RConn1
  PS Switch1/RConn1 -- force/RConn1
  PS Min/LConn2 -- upper_bound/RConn1

== system NUgus_contact/right_foot/foot_br_contact/calculate forces/y contact force ==
  PS Max : fl_lib/Physical Signals/Nonlinear Operators/PS Max
      settings: SourceProductName=Simscape  SourceProductBaseCode=SS
  PS Min : fl_lib/Physical Signals/Nonlinear Operators/PS Min
      settings: SourceProductName=Simscape  SourceProductBaseCode=SS
  PS Switch1 : fl_lib/Physical Signals/Nonlinear Operators/PS Switch  Threshold=0
      settings: SourceProductName=Simscape  SourceProductBaseCode=SS
  frictionless : PMIOPort  Side=Left
  force : PMIOPort  Port=2  Side=Right
  velocity : PMIOPort  Port=3  Side=Left
  z position : PMIOPort  Port=4  Side=Left
  upper_bound : PMIOPort  Port=5  Side=Left
  lower_bound : PMIOPort  Port=6  Side=Left
  connections:
  PS Max/LConn2 -- lower_bound/RConn1
  PS Max/LConn1 -- PS Min/RConn1
  PS Switch1/LConn3 -- PS Max/RConn1
  PS Min/LConn1 -- velocity/RConn1
  z position/RConn1 -- PS Switch1/LConn2
  PS Switch1/LConn1 -- frictionless/RConn1
  PS Switch1/RConn1 -- force/RConn1
  PS Min/LConn2 -- upper_bound/RConn1

== system NUgus_contact/right_foot/foot_fl_contact/calculate forces/x contact force ==
  PS Max : fl_lib/Physical Signals/Nonlinear Operators/PS Max
      settings: SourceProductName=Simscape  SourceProductBaseCode=SS
  PS Min : fl_lib/Physical Signals/Nonlinear Operators/PS Min
      settings: SourceProductName=Simscape  SourceProductBaseCode=SS
  PS Switch1 : fl_lib/Physical Signals/Nonlinear Operators/PS Switch  Threshold=0
      settings: SourceProductName=Simscape  SourceProductBaseCode=SS
  frictionless : PMIOPort  Side=Left
  force : PMIOPort  Port=2  Side=Right
  velocity : PMIOPort  Port=3  Side=Left
  z position : PMIOPort  Port=4  Side=Left
  upper_bound : PMIOPort  Port=5  Side=Left
  lower_bound : PMIOPort  Port=6  Side=Left
  connections:
  PS Max/LConn2 -- lower_bound/RConn1
  PS Max/LConn1 -- PS Min/RConn1
  PS Switch1/LConn3 -- PS Max/RConn1
  PS Min/LConn1 -- velocity/RConn1
  z position/RConn1 -- PS Switch1/LConn2
  PS Switch1/LConn1 -- frictionless/RConn1
  PS Switch1/RConn1 -- force/RConn1
  PS Min/LConn2 -- upper_bound/RConn1

== system NUgus_contact/right_foot/foot_fl_contact/calculate forces/y contact force ==
  PS Max : fl_lib/Physical Signals/Nonlinear Operators/PS Max
      settings: SourceProductName=Simscape  SourceProductBaseCode=SS
  PS Min : fl_lib/Physical Signals/Nonlinear Operators/PS Min
      settings: SourceProductName=Simscape  SourceProductBaseCode=SS
  PS Switch1 : fl_lib/Physical Signals/Nonlinear Operators/PS Switch  Threshold=0
      settings: SourceProductName=Simscape  SourceProductBaseCode=SS
  frictionless : PMIOPort  Side=Left
  force : PMIOPort  Port=2  Side=Right
  velocity : PMIOPort  Port=3  Side=Left
  z position : PMIOPort  Port=4  Side=Left
  upper_bound : PMIOPort  Port=5  Side=Left
  lower_bound : PMIOPort  Port=6  Side=Left
  connections:
  PS Max/LConn2 -- lower_bound/RConn1
  PS Max/LConn1 -- PS Min/RConn1
  PS Switch1/LConn3 -- PS Max/RConn1
  PS Min/LConn1 -- velocity/RConn1
  z position/RConn1 -- PS Switch1/LConn2
  PS Switch1/LConn1 -- frictionless/RConn1
  PS Switch1/RConn1 -- force/RConn1
  PS Min/LConn2 -- upper_bound/RConn1

== system NUgus_contact/right_foot/foot_fr_contact/calculate forces/x contact force ==
  PS Max : fl_lib/Physical Signals/Nonlinear Operators/PS Max
      settings: SourceProductName=Simscape  SourceProductBaseCode=SS
  PS Min : fl_lib/Physical Signals/Nonlinear Operators/PS Min
      settings: SourceProductName=Simscape  SourceProductBaseCode=SS
  PS Switch1 : fl_lib/Physical Signals/Nonlinear Operators/PS Switch  Threshold=0
      settings: SourceProductName=Simscape  SourceProductBaseCode=SS
  frictionless : PMIOPort  Side=Left
  force : PMIOPort  Port=2  Side=Right
  velocity : PMIOPort  Port=3  Side=Left
  z position : PMIOPort  Port=4  Side=Left
  upper_bound : PMIOPort  Port=5  Side=Left
  lower_bound : PMIOPort  Port=6  Side=Left
  connections:
  PS Max/LConn2 -- lower_bound/RConn1
  PS Max/LConn1 -- PS Min/RConn1
  PS Switch1/LConn3 -- PS Max/RConn1
  PS Min/LConn1 -- velocity/RConn1
  z position/RConn1 -- PS Switch1/LConn2
  PS Switch1/LConn1 -- frictionless/RConn1
  PS Switch1/RConn1 -- force/RConn1
  PS Min/LConn2 -- upper_bound/RConn1

== system NUgus_contact/right_foot/foot_fr_contact/calculate forces/y contact force ==
  PS Max : fl_lib/Physical Signals/Nonlinear Operators/PS Max
      settings: SourceProductName=Simscape  SourceProductBaseCode=SS
  PS Min : fl_lib/Physical Signals/Nonlinear Operators/PS Min
      settings: SourceProductName=Simscape  SourceProductBaseCode=SS
  PS Switch1 : fl_lib/Physical Signals/Nonlinear Operators/PS Switch  Threshold=0
      settings: SourceProductName=Simscape  SourceProductBaseCode=SS
  frictionless : PMIOPort  Side=Left
  force : PMIOPort  Port=2  Side=Right
  velocity : PMIOPort  Port=3  Side=Left
  z position : PMIOPort  Port=4  Side=Left
  upper_bound : PMIOPort  Port=5  Side=Left
  lower_bound : PMIOPort  Port=6  Side=Left
  connections:
  PS Max/LConn2 -- lower_bound/RConn1
  PS Max/LConn1 -- PS Min/RConn1
  PS Switch1/LConn3 -- PS Max/RConn1
  PS Min/LConn1 -- velocity/RConn1
  z position/RConn1 -- PS Switch1/LConn2
  PS Switch1/LConn1 -- frictionless/RConn1
  PS Switch1/RConn1 -- force/RConn1
  PS Min/LConn2 -- upper_bound/RConn1
